simulink subsystem "rss_CtlBrdVltgLoLvl1Dia"  (R2023a)
settings: Solver=VariableStepAuto  StartTime=0.0  StopTime=10.0  RelTol=1e-3
undefined symbols (not defined in the file): Cdbl_uCtlBrdVltgMaxVal, ENM_TYPE_FALT, Gu16_ctCtlBrdVltgLoLvl1ConfCnt_C, Gu16_ctCtlBrdVltgLoLvl1RcvyCnt_C, Gu16_uCtlBrdVltgLoLvl1ConfTrs_C, Gu16_uCtlBrdVltgLoLvl1RcvyTrs_C
libraries: vhit_control_library x1, lib_fault_definiteness x1
settings Model: Creator=xiaoqiang.yuan  LastModifiedBy=xiaoqiang.yuan

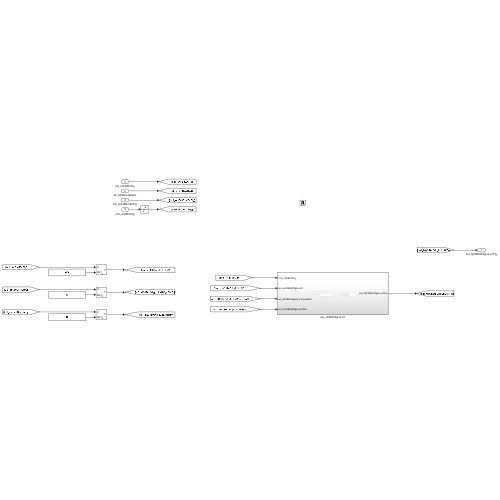
[thumbnail: Simulink's stored preview of the top-level diagram]
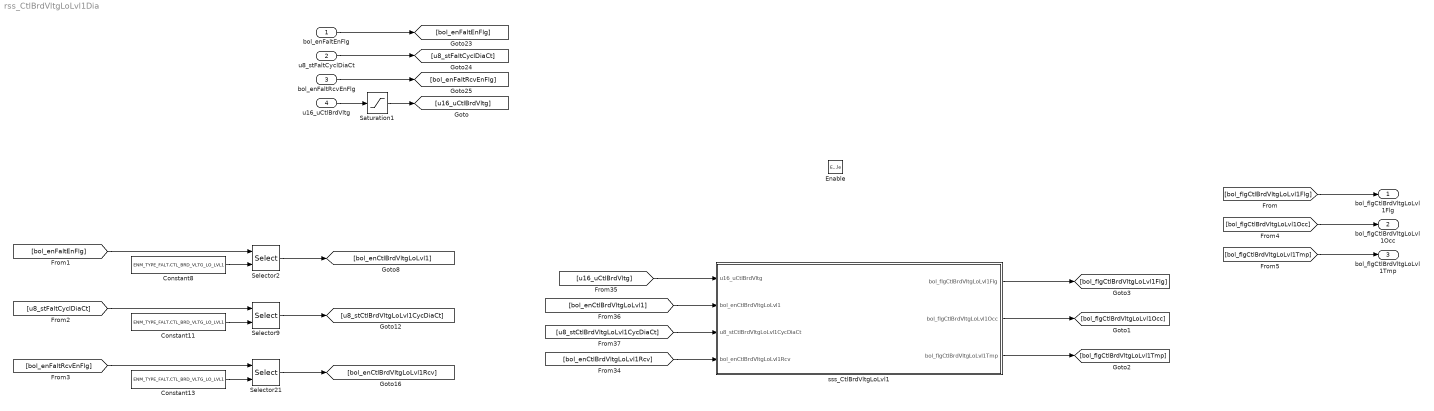
== system rss_CtlBrdVltgLoLvl1Dia ==
  bol_enFaltEnFlg : Inport  OutDataTypeStr=boolean
  u8_stFaltCyclDiaCt : Inport  Port=2  OutDataTypeStr=uint8
  bol_enFaltRcvEnFlg : Inport  Port=3  OutDataTypeStr=boolean
  u16_uCtlBrdVltg : Inport  Port=4  OutDataTypeStr=dt_Standardize_u16p15b0
  Enable : EnablePort
  Constant11 : Constant  Value=ENM_TYPE_FALT.CTL_BRD_VLTG_LO_LVL1
  Constant13 : Constant  Value=ENM_TYPE_FALT.CTL_BRD_VLTG_LO_LVL1
  Constant8 : Constant  Value=ENM_TYPE_FALT.CTL_BRD_VLTG_LO_LVL1
  Saturation1 : Saturate  UpperLimit=Cdbl_uCtlBrdVltgMaxVal  LowerLimit=0
  Selector2 : Selector  IndexMode=Zero-based  InputPortWidth=Cdbl_numFaltDiaNum  IndexOptions=Index vector (port)  Indices=[1 3]  OutputSizes=1
  Selector21 : Selector  IndexMode=Zero-based  InputPortWidth=Cdbl_numFaltDiaNum  IndexOptions=Index vector (port)  Indices=[1 3]  OutputSizes=1
  Selector9 : Selector  IndexMode=Zero-based  InputPortWidth=Cdbl_numFaltDiaNum  IndexOptions=Index vector (port)  Indices=[1 3]  OutputSizes=1
  sss_CtlBrdVltgLoLvl1 : Subsystem
  bol_flgCtlBrdVltgLoLvl1Flg : Outport  OutDataTypeStr=boolean
  bol_flgCtlBrdVltgLoLvl1Occ : Outport  Port=2  OutDataTypeStr=boolean
  bol_flgCtlBrdVltgLoLvl1Tmp : Outport  Port=3  OutDataTypeStr=boolean
  wires:
  [bol_flgCtlBrdVltgLoLvl1Flg] -> bol_flgCtlBrdVltgLoLvl1Flg/1
  [u16_uCtlBrdVltg] -> sss_CtlBrdVltgLoLvl1/1(u16_uCtlBrdVltg)
  [u8_stCtlBrdVltgLoLvl1CycDiaCt] -> sss_CtlBrdVltgLoLvl1/3(u8_stCtlBrdVltgLoLvl1CycDiaCt)
  [bol_enCtlBrdVltgLoLvl1] -> sss_CtlBrdVltgLoLvl1/2(bol_enCtlBrdVltgLoLvl1)
  sss_CtlBrdVltgLoLvl1/1(bol_flgCtlBrdVltgLoLvl1Flg) -> [bol_flgCtlBrdVltgLoLvl1Flg]
  [bol_enCtlBrdVltgLoLvl1Rcv] -> sss_CtlBrdVltgLoLvl1/4(bol_enCtlBrdVltgLoLvl1Rcv)
  u16_uCtlBrdVltg/1 -> Saturation1/1
  u8_stFaltCyclDiaCt/1 -> [u8_stFaltCyclDiaCt]
  bol_enFaltRcvEnFlg/1 -> [bol_enFaltRcvEnFlg]
  bol_enFaltEnFlg/1 -> [bol_enFaltEnFlg]
  [u8_stFaltCyclDiaCt] -> Selector9/1
  [bol_enFaltRcvEnFlg] -> Selector21/1
  [bol_enFaltEnFlg] -> Selector2/1
  Selector21/1 -> [bol_enCtlBrdVltgLoLvl1Rcv]
  Selector9/1 -> [u8_stCtlBrdVltgLoLvl1CycDiaCt]
  Selector2/1 -> [bol_enCtlBrdVltgLoLvl1]
  Constant11/1 -> Selector9/2
  Constant13/1 -> Selector21/2
  Constant8/1 -> Selector2/2
  Saturation1/1 -> [u16_uCtlBrdVltg]
  sss_CtlBrdVltgLoLvl1/2(bol_flgCtlBrdVltgLoLvl1Occ) -> [bol_flgCtlBrdVltgLoLvl1Occ]
  [bol_flgCtlBrdVltgLoLvl1Occ] -> bol_flgCtlBrdVltgLoLvl1Occ/1
  [bol_flgCtlBrdVltgLoLvl1Tmp] -> bol_flgCtlBrdVltgLoLvl1Tmp/1
  sss_CtlBrdVltgLoLvl1/3(bol_flgCtlBrdVltgLoLvl1Tmp) -> [bol_flgCtlBrdVltgLoLvl1Tmp]

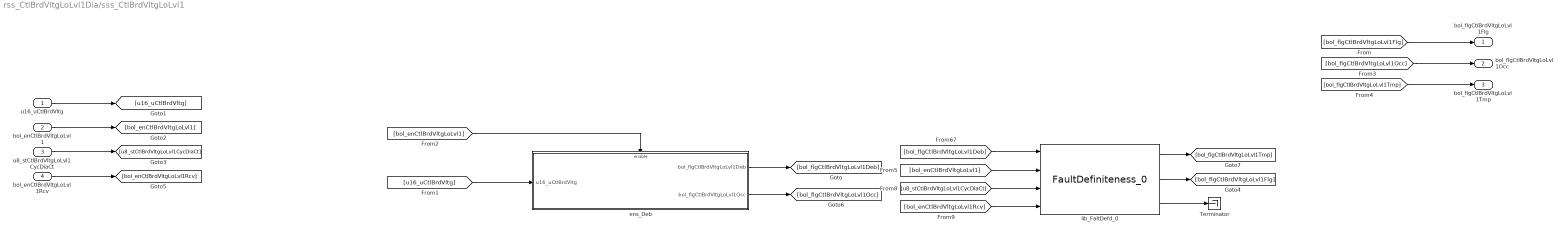
== system rss_CtlBrdVltgLoLvl1Dia/sss_CtlBrdVltgLoLvl1 ==
  u16_uCtlBrdVltg : Inport
  bol_enCtlBrdVltgLoLvl1 : Inport  Port=2
  u8_stCtlBrdVltgLoLvl1CycDiaCt : Inport  Port=3
  bol_enCtlBrdVltgLoLvl1Rcv : Inport  Port=4
  Terminator : Terminator
  ens_Deb : Subsystem
  lib_FaltDefd_0 : lib_fault_definiteness/FaultDefiniteness_0  lb_FaltWaitRecvCnt=Gu16_ctCtlBrdVltgLoLvl1ConfCnt_C
  bol_flgCtlBrdVltgLoLvl1Flg : Outport
  bol_flgCtlBrdVltgLoLvl1Occ : Outport  Port=2
  bol_flgCtlBrdVltgLoLvl1Tmp : Outport  Port=3
  wires:
  [bol_flgCtlBrdVltgLoLvl1Tmp] -> bol_flgCtlBrdVltgLoLvl1Tmp/1
  [bol_flgCtlBrdVltgLoLvl1Occ] -> bol_flgCtlBrdVltgLoLvl1Occ/1
  ens_Deb/2(bol_flgCtlBrdVltgLoLvl1Occ) -> [bol_flgCtlBrdVltgLoLvl1Occ]
  lib_FaltDefd_0/1 -> [bol_flgCtlBrdVltgLoLvl1Tmp]
  lib_FaltDefd_0/2 -> [bol_flgCtlBrdVltgLoLvl1Flg]
  lib_FaltDefd_0/3 -> Terminator/1
  [bol_enCtlBrdVltgLoLvl1] -> ens_Deb/Enable
  [u16_uCtlBrdVltg] -> ens_Deb/1(u16_uCtlBrdVltg)
  ens_Deb/1(bol_flgCtlBrdVltgLoLvl1Deb) -> [bol_flgCtlBrdVltgLoLvl1Deb]
  bol_enCtlBrdVltgLoLvl1Rcv/1 -> [bol_enCtlBrdVltgLoLvl1Rcv]
  u8_stCtlBrdVltgLoLvl1CycDiaCt/1 -> [u8_stCtlBrdVltgLoLvl1CycDiaCt]
  bol_enCtlBrdVltgLoLvl1/1 -> [bol_enCtlBrdVltgLoLvl1]
  [bol_flgCtlBrdVltgLoLvl1Flg] -> bol_flgCtlBrdVltgLoLvl1Flg/1
  u16_uCtlBrdVltg/1 -> [u16_uCtlBrdVltg]
  [bol_enCtlBrdVltgLoLvl1Rcv] -> lib_FaltDefd_0/4
  [u8_stCtlBrdVltgLoLvl1CycDiaCt] -> lib_FaltDefd_0/3
  [bol_enCtlBrdVltgLoLvl1] -> lib_FaltDefd_0/2
  [bol_flgCtlBrdVltgLoLvl1Deb] -> lib_FaltDefd_0/1

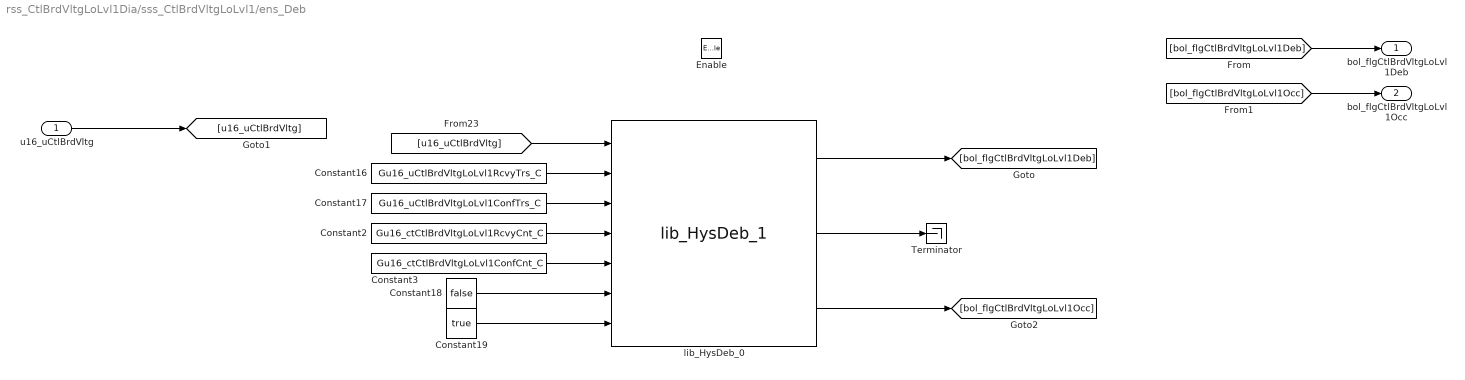
== system rss_CtlBrdVltgLoLvl1Dia/sss_CtlBrdVltgLoLvl1/ens_Deb ==
  u16_uCtlBrdVltg : Inport
  Enable : EnablePort
  Constant16 : Constant  Value=Gu16_uCtlBrdVltgLoLvl1RcvyTrs_C
  Constant17 : Constant  Value=Gu16_uCtlBrdVltgLoLvl1ConfTrs_C
  Constant18 : Constant  Value=false  OutDataTypeStr=boolean
  Constant19 : Constant  Value=true  OutDataTypeStr=boolean
  Constant2 : Constant  Value=Gu16_ctCtlBrdVltgLoLvl1RcvyCnt_C
  Constant3 : Constant  Value=Gu16_ctCtlBrdVltgLoLvl1ConfCnt_C
  Terminator : Terminator
  lib_HysDeb_0 : vhit_control_library/lib_HysDeb_1  lb_parInitOutp=0
  bol_flgCtlBrdVltgLoLvl1Deb : Outport
  bol_flgCtlBrdVltgLoLvl1Occ : Outport  Port=2
  wires:
  [bol_flgCtlBrdVltgLoLvl1Occ] -> bol_flgCtlBrdVltgLoLvl1Occ/1
  lib_HysDeb_0/3 -> [bol_flgCtlBrdVltgLoLvl1Occ]
  lib_HysDeb_0/2 -> Terminator/1
  Constant3/1 -> lib_HysDeb_0/5
  Constant2/1 -> lib_HysDeb_0/4
  Constant19/1 -> lib_HysDeb_0/7
  Constant18/1 -> lib_HysDeb_0/6
  Constant17/1 -> lib_HysDeb_0/3
  Constant16/1 -> lib_HysDeb_0/2
  [u16_uCtlBrdVltg] -> lib_HysDeb_0/1
  u16_uCtlBrdVltg/1 -> [u16_uCtlBrdVltg]
  [bol_flgCtlBrdVltgLoLvl1Deb] -> bol_flgCtlBrdVltgLoLvl1Deb/1
  lib_HysDeb_0/1 -> [bol_flgCtlBrdVltgLoLvl1Deb]
